simulink model "labmaq_F"  (R2023b)
settings: Solver=ode45  StartTime=0.0  StopTime=200  RelTol=1e-3  EnableMultiTasking=on
settings Model: Creator=sergio  LastModifiedBy=klysm
settings DataIOCC: SaveFormat=Array  SignalLoggingSaveFormat=ModelDataLogs  ReturnWorkspaceOutputs=off
settings OptimizationCC: BlockReduction=off  BooleanDataType=off
settings DebuggingCC: SaveWithParameterizedLinksMsg=none  UnderspecifiedInitializationDetection=Classic  MergeDetectMultiDrivingBlocksExec=none  SignalResolutionControl=TryResolveAllWithWarning  MultiTaskDSMMsg=warning  MultiTaskCondExecSysMsg=none  UnconnectedInputMsg=warning  UnconnectedOutputMsg=warning  UnconnectedLineMsg=warning
settings HardwareCC: TargetBitPerPointer=64  TargetBitPerSizeT=64  TargetBitPerPtrDiffT=64  TargetLongLongMode=on  TargetIntDivRoundTo=Zero  TargetEndianess=LittleEndian  TargetWordSize=64  TargetHWDeviceType=MATLAB Host  ProdEqTarget=off
settings ModelReferenceCC: PropagateSignalLabelsOutOfModel=off
settings GRTTargetCC: CombineOutputUpdateFcns=off  GRTInterface=on

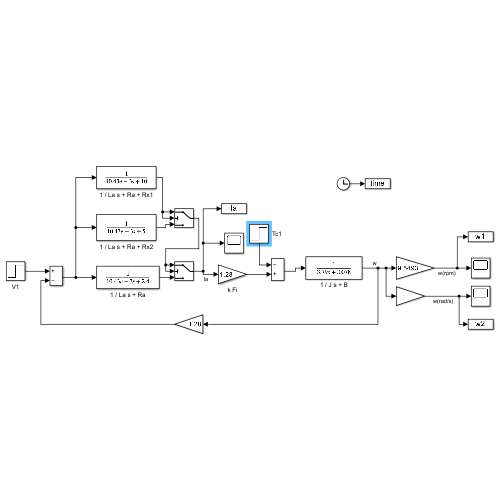
[thumbnail: Simulink's stored preview of the top-level diagram]
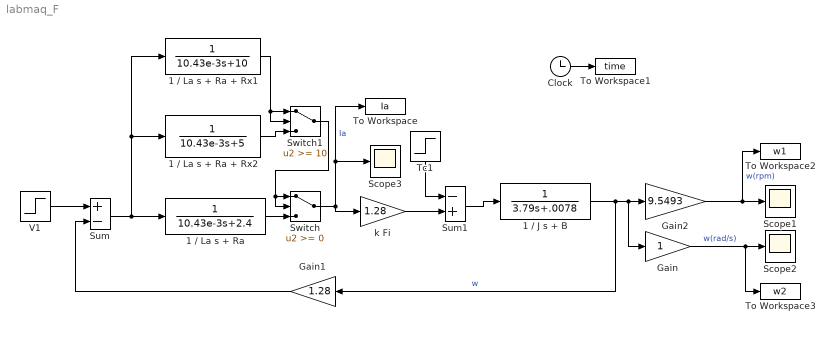
== system labmaq_F ==
  1 / J s + B : TransferFcn  Denominator=[3.79 .0078]
  1 / La s + Ra : TransferFcn  Denominator=[10.43e-3 2.4]
  1 / La s + Ra + Rx1 : TransferFcn  Denominator=[10.43e-3 10]
  1 / La s + Ra + Rx2 : TransferFcn  Denominator=[10.43e-3 5]
  Clock : Clock
  Gain : Gain
  Gain1 : Gain  Gain=1.28  SaturateOnIntegerOverflow=on  OutDataTypeStr=Inherit: Same as input  ParamDataTypeStr=Inherit: Same as input
  Gain2 : Gain  Gain=9.5493  SaturateOnIntegerOverflow=on  OutDataTypeStr=Inherit: Same as input  ParamDataTypeStr=Inherit: Same as input
  Scope1 : Scope
  Scope2 : Scope
  Scope3 : Scope
  Sum : Sum  Inputs=+-  InputSameDT=on  SaturateOnIntegerOverflow=on  OutDataTypeStr=Inherit: Same as first input
  Sum1 : Sum  Inputs=-+  InputSameDT=on  SaturateOnIntegerOverflow=on  OutDataTypeStr=Inherit: Same as first input
  Switch : Switch
  Switch1 : Switch  Threshold=10
  Tc1 : Step  Time=100  After=20  SampleTime=0
  To Workspace : ToWorkspace  VariableName=Ia  SampleTime=-1
  To Workspace1 : ToWorkspace  VariableName=time  SampleTime=-1
  To Workspace2 : ToWorkspace  VariableName=w1  SampleTime=-1
  To Workspace3 : ToWorkspace  VariableName=w2  SampleTime=-1
  V1 : Step  After=220  SampleTime=0
  k Fi : Gain  Gain=1.28  SaturateOnIntegerOverflow=on  OutDataTypeStr=Inherit: Same as input  ParamDataTypeStr=Inherit: Same as input
  wires:
  Sum1/1 -> 1 / J s + B/1
  k Fi/1 -> Sum1/2
  1 / La s + Ra + Rx2/1 -> Switch1/3
  1 / La s + Ra + Rx1/1 -> Switch1/1, Switch1/2
  Switch1/1 -> Switch/1, Switch/2
  Gain1/1 -> Sum/2
  1 / J s + B/1 -> Gain/1, Gain2/1, Gain1/1  "w"
  Gain2/1 -> Scope1/1, To Workspace2/1  "w(rpm)"
  V1/1 -> Sum/1
  Sum/1 -> 1 / La s + Ra + Rx1/1, 1 / La s + Ra + Rx2/1, 1 / La s + Ra/1
  Tc1/1 -> Sum1/1
  1 / La s + Ra/1 -> Switch/3
  Switch/1 -> k Fi/1, Scope3/1, To Workspace/1  "Ia"
  Gain/1 -> Scope2/1, To Workspace3/1  "w(rad/s)"
  Clock/1 -> To Workspace1/1
